simulink model "act1_simulink_sesion2"  (R2020a)
settings: Solver=ode1  StartTime=0.0  StopTime=10.0  FixedStep=0.001  RelTol=1e-3
undefined symbols (not defined in the file or in its folder): a_I, a_II, a_III, b_I, b_II, b_III
settings Model: Creator=Jorjolo  LastModifiedBy=Jorjolo

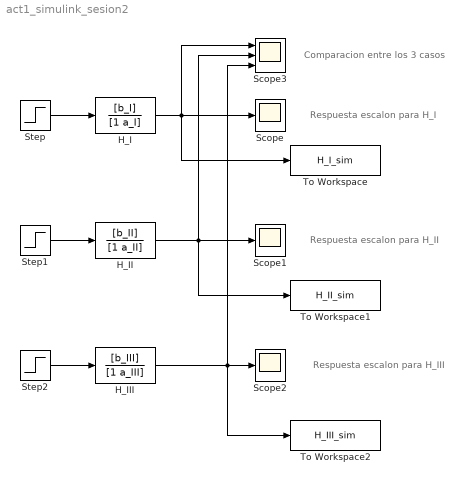
== system act1_simulink_sesion2 ==
  note: Respuesta escalon para H_I
  note: Comparacion entre los 3 casos
  note: Respuesta escalon para H_II
  note: Respuesta escalon para H_III
  H_I : TransferFcn  Numerator=[b_I]  Denominator=[1 a_I]
  H_II : TransferFcn  Numerator=[b_II]  Denominator=[1 a_II]
  H_III : TransferFcn  Numerator=[b_III]  Denominator=[1 a_III]
  Scope : Scope
  Scope1 : Scope
  Scope2 : Scope
  Scope3 : Scope  NumInputPorts=3
  Step : Step  SampleTime=0
  Step1 : Step  SampleTime=0
  Step2 : Step  SampleTime=0
  To Workspace : ToWorkspace  VariableName=H_I_sim  SaveFormat=Timeseries  SampleTime=-1
  To Workspace1 : ToWorkspace  VariableName=H_II_sim  SaveFormat=Timeseries  SampleTime=-1
  To Workspace2 : ToWorkspace  VariableName=H_III_sim  SaveFormat=Timeseries  SampleTime=-1
  wires:
  H_III/1 -> To Workspace2/1, Scope3/3, Scope2/1
  H_II/1 -> To Workspace1/1, Scope3/2, Scope1/1
  Step/1 -> H_I/1
  Step1/1 -> H_II/1
  Step2/1 -> H_III/1
  H_I/1 -> To Workspace/1, Scope3/1, Scope/1
